simulink model "sim_control_adapt_PI_EKF"  (R2021b)
settings: Solver=ode1  StartTime=0.0  StopTime=120  FixedStep=0.01  RelTol=1e-3
settings Model: PacingRate=3  Creator=ONLY-GOD  LastModifiedBy=ASUS
settings SolverCC: AlgebraicLoopSolver=TrustRegion
settings DebuggingCC: SFMachineParentedDataDiag=warning

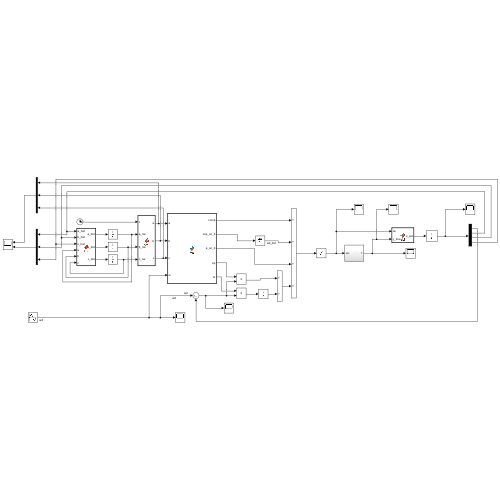
[thumbnail: Simulink's stored preview of the top-level diagram]
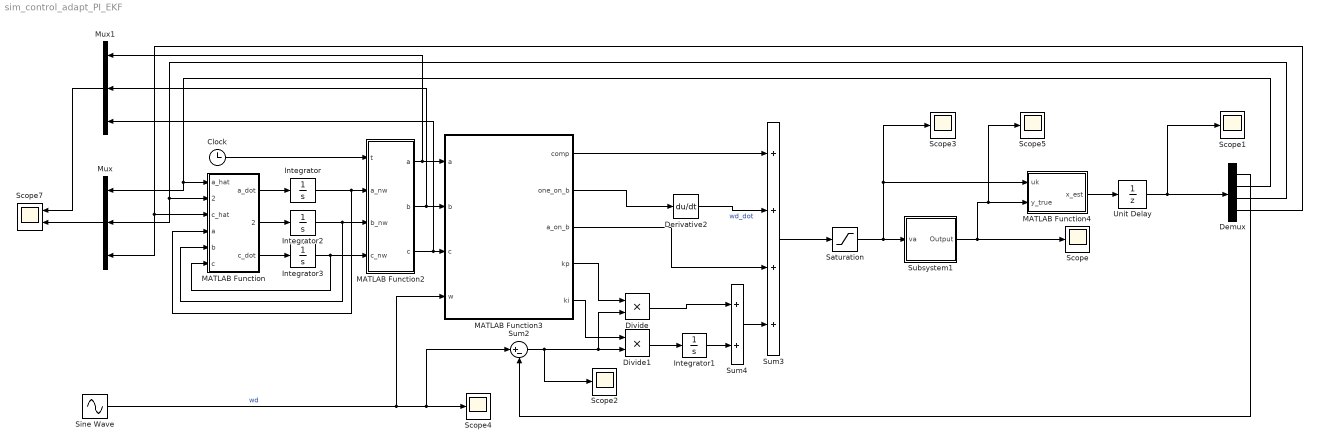
== system sim_control_adapt_PI_EKF ==
  Clock : Clock
  Demux : Demux
  Derivative2 : Derivative
  Divide : Product  Inputs=**
  Divide1 : Product  Inputs=**
  Integrator : Integrator  InitialCondition=27.65
  Integrator1 : Integrator
  Integrator2 : Integrator  InitialCondition=17.35
  Integrator3 : Integrator  InitialCondition=5.635
  MATLAB Function : MATLAB Function  TreatAsAtomicUnit=on
  MATLAB Function2 : MATLAB Function  TreatAsAtomicUnit=on
  MATLAB Function3 : MATLAB Function  TreatAsAtomicUnit=on
  MATLAB Function4 : MATLAB Function  TreatAsAtomicUnit=on
  Mux : Mux  Inputs=3
  Mux1 : Mux  Inputs=3
  Saturation : Saturate  UpperLimit=23  LowerLimit=-23
  Scope{,1..5} (6 alike) : Scope
  Scope7 : Scope  NumInputPorts=2
  Sine Wave : Sin  Amplitude=10  Frequency=2*pi*0.4  SampleTime=0
  Subsystem1 : Subsystem
  Sum2 : Sum  Inputs=|+-
  Sum3 : Sum  Inputs=++++
  Sum4 : Sum
  Unit Delay : UnitDelay  SampleTime=-1  HasFrameUpgradeWarning=on
  wires:
  Derivative2/1 -> Sum3/2  "wd_dot"
  MATLAB Function3/2(one_on_b) -> Derivative2/1
  MATLAB Function3/1(comp) -> Sum3/1
  MATLAB Function3/3(a_on_b) -> Sum3/3
  Sum4/1 -> Sum3/4
  MATLAB Function2/1(a) -> Mux1/1, MATLAB Function3/1(a)
  MATLAB Function2/2(b) -> Mux1/2, MATLAB Function3/2(b)
  MATLAB Function2/3(c) -> Mux1/3, MATLAB Function3/3(c)
  Subsystem1/1(Output) -> Scope/1, Scope5/1, MATLAB Function4/2(y_true)
  MATLAB Function3/4(kp) -> Divide/1
  MATLAB Function3/5(ki) -> Divide1/1
  Sum2/1 -> Scope2/1, Divide/2, Divide1/2
  MATLAB Function4/1(x_est) -> Unit Delay/1
  Divide1/1 -> Integrator1/1
  Integrator1/1 -> Sum4/2
  Divide/1 -> Sum4/1
  Demux/2 -> Mux/1, MATLAB Function/1(a_hat)
  Demux/3 -> Mux/2, MATLAB Function/2(b_hat)
  Demux/4 -> Mux/3, MATLAB Function/3(c_hat)
  Clock/1 -> MATLAB Function2/1(t)
  Sum3/1 -> Saturation/1
  Unit Delay/1 -> Scope1/1, Demux/1
  Sine Wave/1 -> MATLAB Function3/4(w), Sum2/1, Scope4/1  "wd"
  Mux/1 -> Scope7/2
  Saturation/1 -> Scope3/1, MATLAB Function4/1(uk), Subsystem1/1(va)
  Demux/1 -> Sum2/2
  MATLAB Function/1(a_dot) -> Integrator/1
  Integrator/1 -> MATLAB Function2/2(a_nw), MATLAB Function/4(a)
  MATLAB Function/2(b_dot) -> Integrator2/1
  MATLAB Function/3(c_dot) -> Integrator3/1
  Integrator2/1 -> MATLAB Function/5(b), MATLAB Function2/3(b_nw)
  Integrator3/1 -> MATLAB Function2/4(c_nw), MATLAB Function/6(c)
  Mux1/1 -> Scope7/1

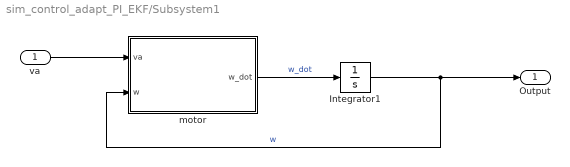
== system sim_control_adapt_PI_EKF/Subsystem1 ==
  va : Inport
  Integrator1 : Integrator
  motor : MATLAB Function  TreatAsAtomicUnit=on
  Output : Outport
  wires:
  Integrator1/1 -> motor/2(w), Output/1  "w"
  motor/1(w_dot) -> Integrator1/1  "w_dot"
  va/1 -> motor/1(va)

== matlab function sim_control_adapt_PI_EKF/MATLAB Function4 ==
  settings: updateMethod=DISCRETE
  data: uk input; y_true input; x_est output
function x_est = ekf(uk,y_true)
Ts = 0.01;
persistent x_est_p P Qd_est R_est Qc_est;
if isempty(x_est_p)
    x_est_p = [0;0;0;0];
    P       = 1e-4*diag([10,1,30,10]);
    Qc_est  = 1e-4*diag([1,10,100,10]);
    Qd_est  = Ts*Qc_est;
    R_est   = 0.001;
end
c  = [1 0 0 0];
D  = 0;
Ck = c;
Dk = D;

%Comput Kalman Gain and update predicted value
Wk    = P*Ck'/(Ck*P*Ck'+R_est);
y_est = Ck*x_est_p+Dk*uk;
x     = x_est_p+Wk.*(y_true-y_est);

%Compute prediction at next time step
x_est = x+Ts*[-x(2)*x(1)+uk*x(3)-x(4)*sign(x(1));
                          0;
                          0;
                          0];

%Update error covariance matrices
P = P-Wk*Ck*P;

%Define Ak
Ak      = eye(4)+Ts*[-x(2) -x(1) uk -sign(x(1));
                 0     0    0      0;
                 0     0    0      0;
                 0     0    0      0];
P       = Ak*P*Ak'+Qd_est;
x_est_p = x_est;

== matlab function sim_control_adapt_PI_EKF/MATLAB Function3 ==
  data: comp output; one_on_b output; a input; a_on_b output; b input; c input; w input; kp output; ki output
function [comp,one_on_b,a_on_b,kp,ki] = fcn(a,b,c,w)

a_on_b = (a/b)*w;
one_on_b = (1/b)*w;
comp = (c/b)*sign(w);

wn = 2*pi*6;
zeta = 1;

ki = wn^2/b;
kp = (2*zeta*wn-a)/b;

== matlab function sim_control_adapt_PI_EKF/MATLAB Function ==
  data: a_hat input; a_dot output; b_hat input; c_hat input; b_dot output; c_dot output; a input; b input; c input
function [a_dot,b_dot,c_dot] = fcn(a_hat,b_hat,c_hat,a,b,c)

lamda = 5;

a_dot = (1/lamda)*(-a+a_hat);
b_dot = (1/lamda)*(-b+b_hat);
c_dot = (1/lamda)*(-c+c_hat);

== matlab function sim_control_adapt_PI_EKF/MATLAB Function2 ==
  data: a output; b output; c output; t input; a_nw input; b_nw input; c_nw input
function [a,b,c] = fcn(t,a_nw,b_nw,c_nw)

a = 27.65;
b = 17.35;
c = 5.635;

if t>40
a = a_nw;
b = b_nw;
c = c_nw;
end

== matlab function sim_control_adapt_PI_EKF/Subsystem1/motor ==
  data: va input; w_dot output; w input
function w_dot = fcn(va, w)
a = 27.65;
b = 17.35;
c = 5.635;

w_dot = -a*w+b*va-c*sign(w);
